simulink model "observador_mejorado"  (R2020a)
settings: Solver=ode45  StartTime=0.0  StopTime=25  MaxStep=1e-4  RelTol=1e-5
model workspace: external: MATLAB File D:\Ferran\Facultad\UNCuyo\Meca\Automática y Máquinas Eléctricas\Proyecto final\matlab2\parametros_y_especs\parametros_y_especif.m (data not in the file)
undefined symbols (not defined in the file): alpha_Cu, Ba, beq, Cts, Jeq, Ke_int, Ke_theta, Ke_theta_m, Ke_w, Ke_w_m, Ksa, Ksia, L_ls, lambda_m, Ld, Lq, Pp, r, R0, Rd, Rq, Rref, Rts_amb, sigbuilder_block, Tref
settings Model: Creator=Ferran  LastModifiedBy=Ferran

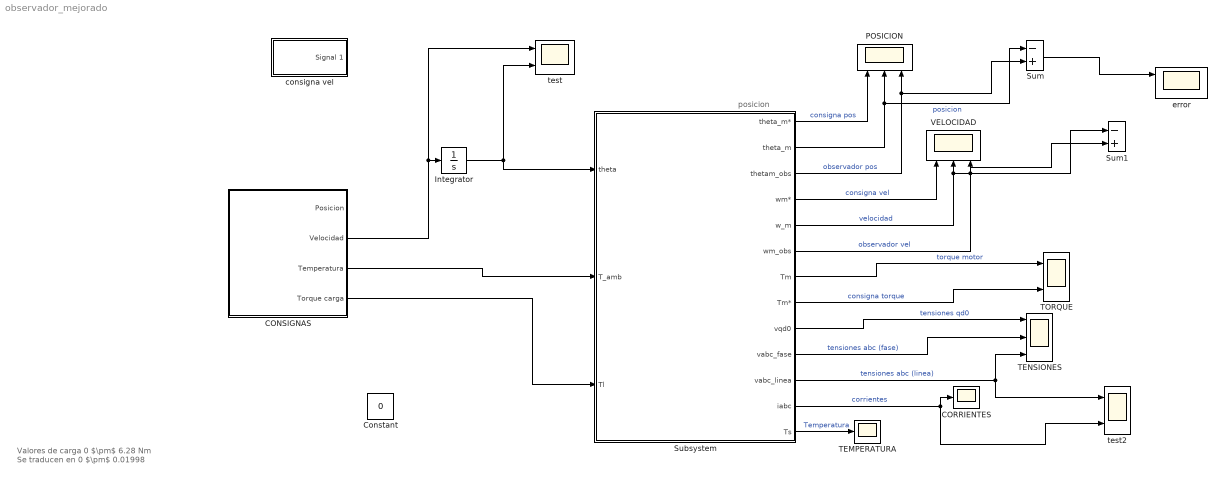
== system observador_mejorado ==
  note: posicion
  note: Valores de carga
      |
      | 0 $\pm$ 6.28 Nm
      | Se traducen en
      | 0 $\pm$ 0.01998
  CONSIGNAS : Subsystem  Tag=STV Subsys  LoadFcn=sigbuilder_block('load');  StartFcn=sigbuilder_block('start');  StopFcn=sigbuilder_block('stop');  ClipboardFcn=sigbuilder_block('clipboard');  mask(Sigbuilder block){tuvar=[0:10]}
      mask help: Simulink:masks:SigbuilderBlock_MD
      mask init:
      | if ~strcmp(get_param(bdroot(gcbh),'SimulationStatus'),'stopped') tuvar = sigbuilder_block('maskInit'); end
      settings: CopyFcn=sigbuilder_block('copy');  DeleteFcn=sigbuilder_block('delete');  ModelCloseFcn=sigbuilder_block('modelClose');  PreSaveFcn=sigbuilder_block('preSave');  PauseFcn=sigbuilder_block('pause');  ContinueFcn=sigbuilder_block('continue');  NameChangeFcn=sigbuilder_block('namechange');  OpenFcn=sigbuilder_block('open',[75 32.4 967.2 484.8 ]);  CloseFcn=sigbuilder_block('close');
      mask Display: plot(0, 0, 100, 100,[2, 2, 32, 32, 2], [68, 8, 8, 68, 68],[32, 2], [38, 38], [32, 19, 2],[53, 60, 44], [32, 17, 17, 2],[16, 16, 31, 31]);txt = getActiveGroup(gcbh);text(2, 100, txt,'verticalAlignment', 'top');
  CORRIENTES : Scope
  Constant : Constant  Value=0
  Integrator : Integrator
  POSICION : Scope  NumInputPorts=3
  Subsystem : Subsystem
  Sum : Sum  Inputs=-+
  Sum1 : Sum  Inputs=-+
  TEMPERATURA : Scope
  TENSIONES : Scope  NumInputPorts=3
  TORQUE : Scope  NumInputPorts=2
  VELOCIDAD : Scope  NumInputPorts=3
  consigna vel : Subsystem  Tag=STV Subsys  LoadFcn=sigbuilder_block('load');  StartFcn=sigbuilder_block('start');  StopFcn=sigbuilder_block('stop');  ClipboardFcn=sigbuilder_block('clipboard');  mask(Sigbuilder block){tuvar=[0:10]}
      mask help: Simulink:masks:SigbuilderBlock_MD
      mask init:
      | if ~strcmp(get_param(bdroot(gcbh),'SimulationStatus'),'stopped') tuvar = sigbuilder_block('maskInit'); end
      settings: CopyFcn=sigbuilder_block('copy');  DeleteFcn=sigbuilder_block('delete');  ModelCloseFcn=sigbuilder_block('modelClose');  PreSaveFcn=sigbuilder_block('preSave');  PauseFcn=sigbuilder_block('pause');  ContinueFcn=sigbuilder_block('continue');  NameChangeFcn=sigbuilder_block('namechange');  OpenFcn=sigbuilder_block('open',[5.4 0 1141.2 552.6 ]);  CloseFcn=sigbuilder_block('close');
      mask Display: plot(0, 0, 100, 100,[2, 2, 32, 32, 2], [68, 8, 8, 68, 68],[32, 2], [38, 38], [32, 19, 2],[53, 60, 44], [32, 17, 17, 2],[16, 16, 31, 31]);txt = getActiveGroup(gcbh);text(2, 100, txt,'verticalAlignment', 'top');
  error : Scope  NumInputPorts=2
  test : Scope  NumInputPorts=2
  test2 : Scope  NumInputPorts=2
  wires:
  CONSIGNAS/3(Temperatura) -> Subsystem/2(T_amb)
  Subsystem/2(theta_m) -> POSICION/2, Sum/1  "posicion"
  Subsystem/1(theta_m*) -> POSICION/1  "consigna pos"
  Subsystem/3(thetam_obs) -> POSICION/3, Sum/2  "observador pos"
  Subsystem/5(w_m) -> Sum1/1, VELOCIDAD/2  "velocidad"
  Subsystem/4(wm*) -> VELOCIDAD/1  "consigna vel"
  Subsystem/6(wm_obs) -> Sum1/2, VELOCIDAD/3  "observador vel"
  Subsystem/7(Tm) -> TORQUE/1  "torque motor"
  Subsystem/8(Tm*) -> TORQUE/2  "consigna torque"
  Subsystem/9(vqd0) -> TENSIONES/1  "tensiones qd0"
  Subsystem/10(vabc_fase) -> TENSIONES/2  "tensiones abc (fase)"
  Subsystem/12(iabc) -> CORRIENTES/1, test2/2  "corrientes"
  Subsystem/13(Ts) -> TEMPERATURA/1  "Temperatura"
  CONSIGNAS/2(Velocidad) -> test/1, Integrator/1
  Subsystem/11(vabc_linea) -> TENSIONES/3, test2/1  "tensiones abc (linea)"
  Integrator/1 -> test/2, Subsystem/1(theta)
  CONSIGNAS/4(Torque carga) -> Subsystem/3(Tl)
  Sum/1 -> error/1

== system observador_mejorado/CONSIGNAS ==
  Demux : Demux  Tag=STV Demux
      settings: DisplayOption=none
  FromWs : FromWorkspace  Tag=STV FromWs  VariableName=tuvar
      SigBuilderData=|
      | common.afterFinalStr = 'Extrapolate'
      | common.sampleTime = 0
      | dataSet.timeRange = [0 25]
      | dataSet.name = 'Group 1'
      | sbobj.Groups.Name = 'Group 1'
      | sbobj.Groups.Signals(1).Name = 'Posicion'
      | sbobj.Groups.Signals(1).XData = [0 5 10 15 20 25]
      | sbobj.Groups.Signals(1).YData = [0 0 6.28318530718 6.28318530718 0 0]
      | sbobj.Groups.Signals(2).Name = 'Velocidad'
      | sbobj.Groups.Signals(2).XData = [0 5 5.25 9.75 10 15 15.25 19.75 20 25]
      | sbobj.Groups.Signals(2).YData = [0 0 1.3228 1.3228 0 0 -1.3228 -1.3228 0 0]
      | sbobj.Groups.Signals(3).Name = 'Temperatura'
      | sbobj.Groups.Signals(3).XData = [0 25]
      | sbobj.Groups.Signals(3).YData = [40 40]
      | sbobj.Groups.Signals(4).Name = 'Torque carga'
      | sbobj.Groups.Signals(4).XData = [0 12.5 12.5 25]
      | sbobj.Groups.Signals(4).YData = [0 0 6.28 6.28]
      | sbobj.Groups.TimeRange = [0 25]
  Posicion : Outport  Tag=STV Outport
  Velocidad : Outport  Tag=STV Outport  Port=2
  Temperatura : Outport  Tag=STV Outport  Port=3
  Torque carga : Outport  Tag=STV Outport  Port=4
  wires:
  FromWs/1 -> Demux/1
  Demux/1 -> Posicion/1
  Demux/2 -> Velocidad/1
  Demux/3 -> Temperatura/1
  Demux/4 -> Torque carga/1

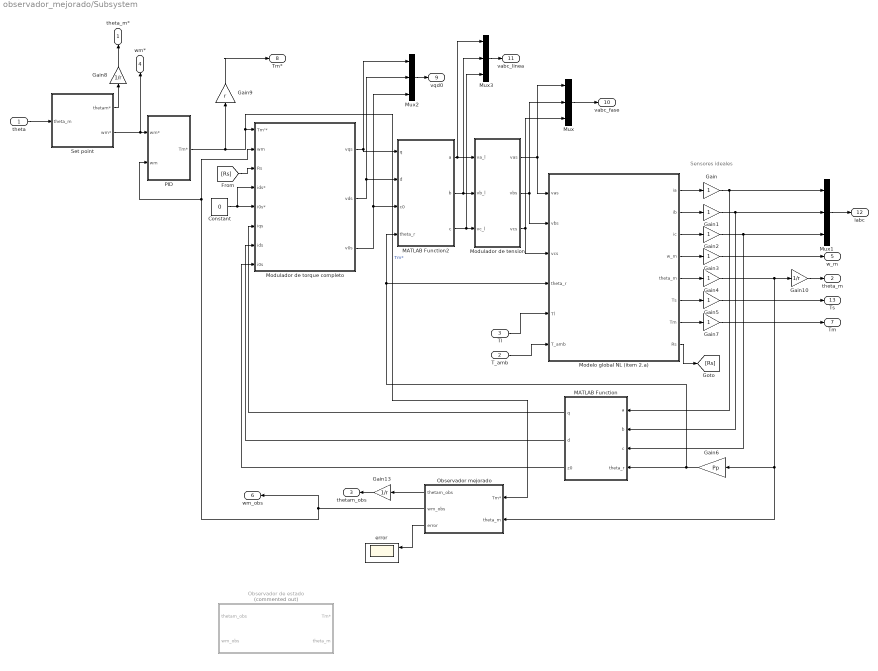
== system observador_mejorado/Subsystem ==
  note: Sensores ideales
  theta : Inport
  T_amb : Inport  Port=2
  Tl : Inport  Port=3
  Constant : Constant  Value=0
  Gain{,1..5,7} (7 alike) : Gain
  Gain10 : Gain  Gain=1/r
  Gain13 : Gain  Gain=1/r
  Gain6 : Gain  Gain=Pp
  Gain8 : Gain  Gain=1/r
  Gain9 : Gain  Gain=r
  MATLAB Function : MATLAB Function  TreatAsAtomicUnit=on
  MATLAB Function2 : MATLAB Function  TreatAsAtomicUnit=on
  Modelo global NL (item 2.a) : Subsystem
  Modulador de tension : Subsystem
  Modulador de torque completo : Subsystem
  Mux{,1..3} (4 alike) : Mux  Inputs=3
  Observador de estado : Subsystem  Commented=on
  Observador mejorado : Subsystem
  PID : Subsystem
  Set point : Subsystem
  error : Scope  NumInputPorts=2
  theta_m* : Outport
  theta_m : Outport  Port=2
  thetam_obs : Outport  Port=3
  wm* : Outport  Port=4
  w_m : Outport  Port=5
  wm_obs : Outport  Port=6
  Tm : Outport  Port=7
  Tm* : Outport  Port=8
  vqd0 : Outport  Port=9
  vabc_fase : Outport  Port=10
  vabc_linea : Outport  Port=11
  iabc : Outport  Port=12
  Ts : Outport  Port=13
  wires:
  Gain4/1 -> Gain10/1, Observador mejorado/2(theta_m), Gain6/1
  Gain1/1 -> Mux1/2, MATLAB Function/2(b)
  Gain/1 -> Mux1/1, MATLAB Function/1(a)
  Gain6/1 -> Modelo global NL (item 2.a)/4(theta_r), MATLAB Function2/4(theta_r), MATLAB Function/4(theta_r)
  MATLAB Function2/3(c) -> Modulador de tension/3(vc_l), Mux3/3
  Modelo global NL (item 2.a)/2(ib) -> Gain1/1
  Observador mejorado/1(thetam_obs) -> Gain13/1
  Modulador de torque completo/1(vqs) -> MATLAB Function2/1(q), Mux2/1
  Set point/1(thetam*) -> Gain8/1
  T_amb/1 -> Modelo global NL (item 2.a)/6(T_amb)
  MATLAB Function/3(z0) -> Modulador de torque completo/8(i0s)
  theta/1 -> Set point/1(theta_m)
  Modulador de tension/2(vbs) -> Modelo global NL (item 2.a)/2(vbs), Mux/2
  Modelo global NL (item 2.a)/5(theta_m) -> Gain4/1
  Modulador de tension/1(vas) -> Modelo global NL (item 2.a)/1(vas), Mux/1
  Tl/1 -> Modelo global NL (item 2.a)/5(Tl)
  Modelo global NL (item 2.a)/4(w_m) -> Gain3/1
  Modelo global NL (item 2.a)/1(ia) -> Gain/1
  Constant/1 -> Modulador de torque completo/4(ids*), Modulador de torque completo/5(i0s*)
  Gain2/1 -> Mux1/3, MATLAB Function/3(c)
  MATLAB Function/2(d) -> Modulador de torque completo/7(ids)
  Modulador de torque completo/2(vds) -> Mux2/2, MATLAB Function2/2(d)
  Gain7/1 -> Tm/1
  MATLAB Function/1(q) -> Modulador de torque completo/6(iqs)
  [Rs] -> Modulador de torque completo/3(Rs)
  Modulador de torque completo/3(v0s) -> Mux2/3, MATLAB Function2/3(c0)
  Gain5/1 -> Ts/1
  Modulador de tension/3(vcs) -> Modelo global NL (item 2.a)/3(vcs), Mux/3
  PID/1(Tm*) -> Gain9/1, Observador mejorado/1(Tm*), Modulador de torque completo/1(Tm'*)  "Tm*"
  Modelo global NL (item 2.a)/6(Ts) -> Gain5/1
  MATLAB Function2/2(b) -> Modulador de tension/2(vb_l), Mux3/2
  Modelo global NL (item 2.a)/3(ic) -> Gain2/1
  MATLAB Function2/1(a) -> Modulador de tension/1(va_l), Mux3/1
  Modelo global NL (item 2.a)/8(Rs) -> [Rs]
  Mux/1 -> vabc_fase/1
  Mux1/1 -> iabc/1
  Mux2/1 -> vqd0/1
  Modelo global NL (item 2.a)/7(Tm) -> Gain7/1
  Gain8/1 -> theta_m*/1
  Set point/2(wm*) -> wm*/1, PID/1(wm*)
  Gain3/1 -> w_m/1
  Gain10/1 -> theta_m/1
  Observador mejorado/2(wm_obs) -> Modulador de torque completo/2(wm), PID/2(wm), wm_obs/1
  Gain13/1 -> thetam_obs/1
  Gain9/1 -> Tm*/1
  Mux3/1 -> vabc_linea/1
  Observador mejorado/3(error) -> error/1

== system observador_mejorado/consigna vel ==
  Demux : Demux  Tag=STV Demux  Outputs=1
      settings: DisplayOption=none
  FromWs : FromWorkspace  Tag=STV FromWs  VariableName=tuvar
      SigBuilderData=|
      | common.afterFinalStr = 'Extrapolate'
      | common.sampleTime = 0
      | dataSet.timeRange = [0 25]
      | dataSet.name = 'Group 1'
      | sbobj.Groups.Name = 'Group 1'
      | sbobj.Groups.Signals.Name = 'Signal 1'
      | sbobj.Groups.Signals.XData = [0 5 7.5 10 15 16.25 18.75 20 25]
      | sbobj.Groups.Signals.YData = [0 0 1.68 0 0 -1.68 -1.68 0 0]
      | sbobj.Groups.TimeRange = [0 25]
  Signal 1 : Outport  Tag=STV Outport
  wires:
  Demux/1 -> Signal 1/1
  FromWs/1 -> Demux/1

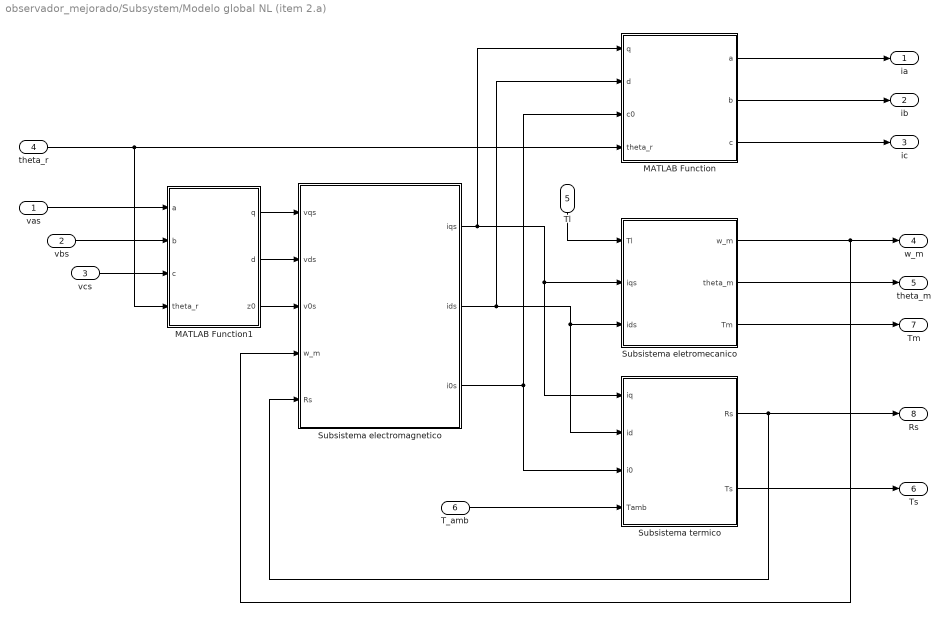
== system observador_mejorado/Subsystem/Modelo global NL (item 2.a) ==
  vas : Inport
  vbs : Inport  Port=2
  vcs : Inport  Port=3
  theta_r : Inport  Port=4
  Tl : Inport  Port=5
  T_amb : Inport  Port=6
  MATLAB Function : MATLAB Function  TreatAsAtomicUnit=on
  MATLAB Function1 : MATLAB Function  TreatAsAtomicUnit=on
  Subsistema electromagnetico : Subsystem
  Subsistema eletromecanico : Subsystem
  Subsistema termico : Subsystem
  ia : Outport
  ib : Outport  Port=2
  ic : Outport  Port=3
  w_m : Outport  Port=4
  theta_m : Outport  Port=5
  Ts : Outport  Port=6
  Tm : Outport  Port=7
  Rs : Outport  Port=8
  wires:
  Subsistema eletromecanico/1(w_m) -> Subsistema electromagnetico/4(w_m), w_m/1
  MATLAB Function1/1(q) -> Subsistema electromagnetico/1(vqs)
  Subsistema eletromecanico/2(theta_m) -> theta_m/1
  MATLAB Function/1(a) -> ia/1
  MATLAB Function/2(b) -> ib/1
  MATLAB Function1/2(d) -> Subsistema electromagnetico/2(vds)
  Subsistema electromagnetico/2(ids) -> Subsistema termico/2(id), Subsistema eletromecanico/3(ids), MATLAB Function/2(d)
  Tl/1 -> Subsistema eletromecanico/1(Tl)
  Subsistema termico/2(Ts) -> Ts/1
  Subsistema electromagnetico/3(i0s) -> Subsistema termico/3(i0), MATLAB Function/3(c0)
  Subsistema termico/1(Rs) -> Subsistema electromagnetico/5(Rs), Rs/1
  vbs/1 -> MATLAB Function1/2(b)
  vcs/1 -> MATLAB Function1/3(c)
  Subsistema electromagnetico/1(iqs) -> Subsistema termico/1(iq), Subsistema eletromecanico/2(iqs), MATLAB Function/1(q)
  vas/1 -> MATLAB Function1/1(a)
  MATLAB Function1/3(z0) -> Subsistema electromagnetico/3(v0s)
  MATLAB Function/3(c) -> ic/1
  Subsistema eletromecanico/3(Tm) -> Tm/1
  theta_r/1 -> MATLAB Function/4(theta_r), MATLAB Function1/4(theta_r)
  T_amb/1 -> Subsistema termico/4(Tamb)

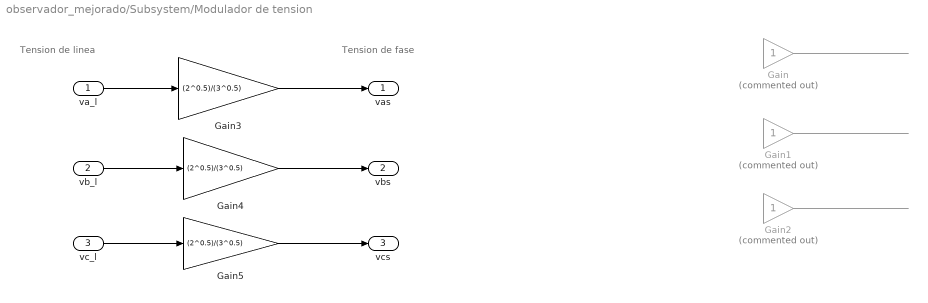
== system observador_mejorado/Subsystem/Modulador de tension ==
  note: Tension de fase
  note: Tension de linea
  va_l : Inport
  vb_l : Inport  Port=2
  vc_l : Inport  Port=3
  Gain : Gain  Commented=on
  Gain1 : Gain  Commented=on
  Gain2 : Gain  Commented=on
  Gain3 : Gain  Gain=(2^0.5)/(3^0.5)
  Gain4 : Gain  Gain=(2^0.5)/(3^0.5)
  Gain5 : Gain  Gain=(2^0.5)/(3^0.5)
  vas : Outport
  vbs : Outport  Port=2
  vcs : Outport  Port=3
  wires:
  Gain4/1 -> vbs/1
  Gain3/1 -> vas/1
  va_l/1 -> Gain3/1
  vb_l/1 -> Gain4/1
  vc_l/1 -> Gain5/1
  Gain5/1 -> vcs/1
  Gain1/1 -> ?
  ? -> Gain/1
  ? -> Gain2/1
  Gain2/1 -> ?
  ? -> Gain1/1
  Gain/1 -> ?

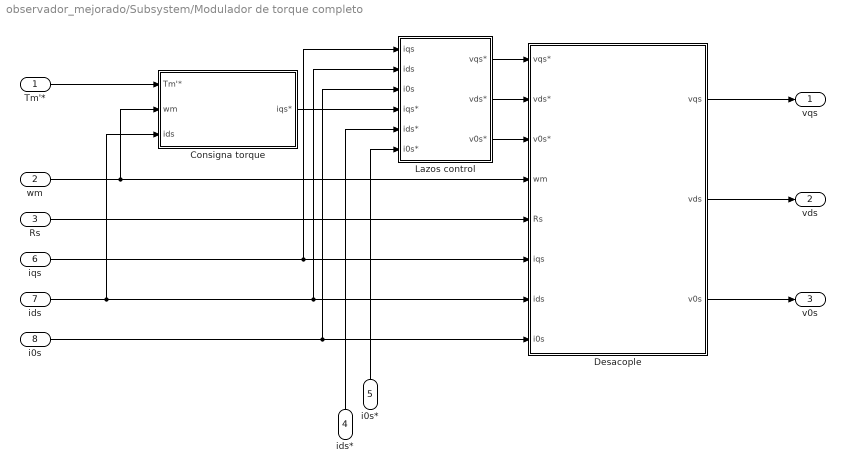
== system observador_mejorado/Subsystem/Modulador de torque completo ==
  Tm'* : Inport
  wm : Inport  Port=2
  Rs : Inport  Port=3
  ids* : Inport  Port=4
  i0s* : Inport  Port=5
  iqs : Inport  Port=6
  ids : Inport  Port=7
  i0s : Inport  Port=8
  Consigna torque : Subsystem
  Desacople : Subsystem
  Lazos control : Subsystem
  vqs : Outport
  vds : Outport  Port=2
  v0s : Outport  Port=3
  wires:
  ids/1 -> Consigna torque/3(ids), Desacople/7(ids), Lazos control/2(ids)
  Lazos control/3(v0s*) -> Desacople/3(v0s*)
  Rs/1 -> Desacople/5(Rs)
  Lazos control/1(vqs*) -> Desacople/1(vqs*)
  wm/1 -> Consigna torque/2(wm), Desacople/4(wm)
  i0s*/1 -> Lazos control/6(i0s*)
  Lazos control/2(vds*) -> Desacople/2(vds*)
  Consigna torque/1(iqs*) -> Lazos control/4(iqs*)
  i0s/1 -> Desacople/8(i0s), Lazos control/3(i0s)
  Desacople/2(vds) -> vds/1
  Tm'*/1 -> Consigna torque/1(Tm'*)
  iqs/1 -> Desacople/6(iqs), Lazos control/1(iqs)
  ids*/1 -> Lazos control/5(ids*)
  Desacople/3(v0s) -> v0s/1
  Desacople/1(vqs) -> vqs/1

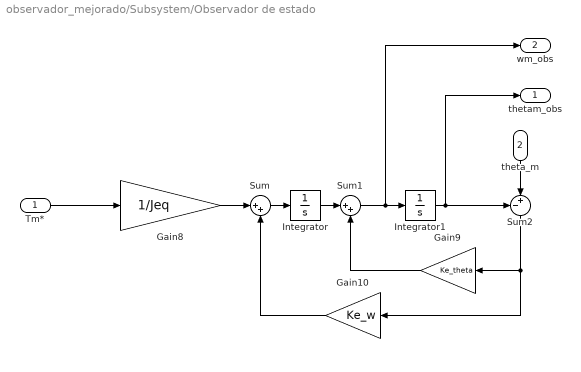
== system observador_mejorado/Subsystem/Observador de estado ==
  Tm* : Inport
  theta_m : Inport  Port=2
  Gain10 : Gain  Gain=Ke_w
  Gain8 : Gain  Gain=1/Jeq
  Gain9 : Gain  Gain=Ke_theta
  Integrator : Integrator
  Integrator1 : Integrator
  Sum : Sum  Inputs=|++
  Sum1 : Sum  Inputs=|++
  Sum2 : Sum  Inputs=-+|
  thetam_obs : Outport
  wm_obs : Outport  Port=2
  wires:
  Sum/1 -> Integrator/1
  Sum1/1 -> wm_obs/1, Integrator1/1
  Integrator1/1 -> thetam_obs/1, Sum2/1
  Gain9/1 -> Sum1/2
  Tm*/1 -> Gain8/1
  Gain8/1 -> Sum/1
  Integrator/1 -> Sum1/1
  Sum2/1 -> Gain10/1, Gain9/1
  Gain10/1 -> Sum/2
  theta_m/1 -> Sum2/2

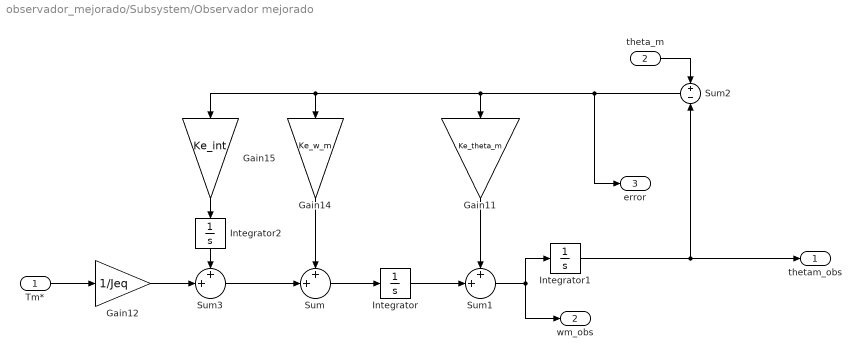
== system observador_mejorado/Subsystem/Observador mejorado ==
  Tm* : Inport
  theta_m : Inport  Port=2
  Gain11 : Gain  Gain=Ke_theta_m
  Gain12 : Gain  Gain=1/Jeq
  Gain14 : Gain  Gain=Ke_w_m
  Gain15 : Gain  Gain=Ke_int
  Integrator : Integrator
  Integrator1 : Integrator
  Integrator2 : Integrator
  Sum : Sum  Inputs=++|
  Sum1 : Sum  Inputs=++|
  Sum2 : Sum  Inputs=+-
  Sum3 : Sum  Inputs=++|
  thetam_obs : Outport
  wm_obs : Outport  Port=2
  error : Outport  Port=3
  wires:
  Sum/1 -> Integrator/1
  Sum1/1 -> wm_obs/1, Integrator1/1
  Integrator/1 -> Sum1/2
  Sum2/1 -> error/1, Gain11/1, Gain14/1, Gain15/1
  Gain12/1 -> Sum3/2
  theta_m/1 -> Sum2/1
  Gain15/1 -> Integrator2/1
  Sum3/1 -> Sum/2
  Gain14/1 -> Sum/1
  Tm*/1 -> Gain12/1
  Integrator1/1 -> thetam_obs/1, Sum2/2
  Gain11/1 -> Sum1/1
  Integrator2/1 -> Sum3/1

== system observador_mejorado/Subsystem/PID ==
  wm* : Inport
  wm : Inport  Port=2
  Gain10 : Gain  Gain=Ksia
  Gain8 : Gain  Gain=Ba
  Gain9 : Gain  Gain=Ksa
  Integrator : Integrator
  Integrator1 : Integrator
  Sum : Sum  Inputs=|+-
  Sum1 : Sum  Inputs=+++
  Tm* : Outport
  wires:
  Sum/1 -> Gain8/1, Integrator/1
  Gain9/1 -> Sum1/2
  wm*/1 -> Sum/1
  Integrator/1 -> Integrator1/1, Gain9/1
  Gain8/1 -> Sum1/3
  Gain10/1 -> Sum1/1
  wm/1 -> Sum/2
  Integrator1/1 -> Gain10/1
  Sum1/1 -> Tm*/1

== system observador_mejorado/Subsystem/Set point ==
  note: Referencia de posicion articular q
  theta_m : Inport
  Derivative : Derivative
  Gain8 : Gain  Gain=r
  thetam* : Outport
  wm* : Outport  Port=2
  wires:
  Derivative/1 -> wm*/1
  theta_m/1 -> Gain8/1
  Gain8/1 -> thetam*/1, Derivative/1

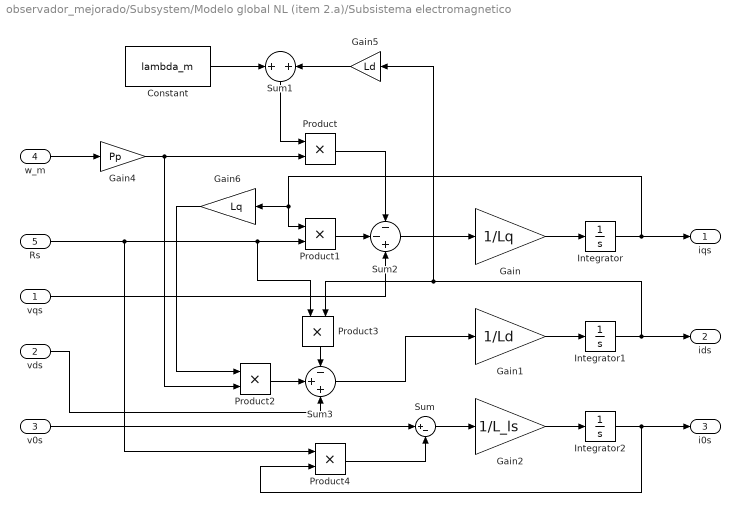
== system observador_mejorado/Subsystem/Modelo global NL (item 2.a)/Subsistema electromagnetico ==
  vqs : Inport
  vds : Inport  Port=2
  v0s : Inport  Port=3
  w_m : Inport  Port=4
  Rs : Inport  Port=5
  Constant : Constant  Value=lambda_m
  Gain : Gain  Gain=1/Lq
  Gain1 : Gain  Gain=1/Ld
  Gain2 : Gain  Gain=1/L_ls
  Gain4 : Gain  Gain=Pp
  Gain5 : Gain  Gain=Ld
  Gain6 : Gain  Gain=Lq
  Integrator : Integrator
  Integrator1 : Integrator
  Integrator2 : Integrator
  Product{,1..4} (5 alike) : Product
  Sum : Sum  Inputs=|+-
  Sum1 : Sum  Inputs=+|+
  Sum2 : Sum  Inputs=--+
  Sum3 : Sum  Inputs=-++
  iqs : Outport
  ids : Outport  Port=2
  i0s : Outport  Port=3
  wires:
  Sum2/1 -> Gain/1
  Integrator1/1 -> ids/1, Product3/2, Gain5/1
  Product1/1 -> Sum2/2
  Integrator/1 -> iqs/1, Gain6/1, Product1/1
  Sum3/1 -> Gain1/1
  Constant/1 -> Sum1/1
  Gain2/1 -> Integrator2/1
  Product3/1 -> Sum3/1
  Gain6/1 -> Product2/1
  Rs/1 -> Product1/2, Product3/1, Product4/1
  v0s/1 -> Sum/1
  w_m/1 -> Gain4/1
  Gain1/1 -> Integrator1/1
  Integrator2/1 -> i0s/1, Product4/2
  vqs/1 -> Sum2/3
  Product4/1 -> Sum/2
  Product2/1 -> Sum3/2
  Gain5/1 -> Sum1/2
  vds/1 -> Sum3/3
  Gain4/1 -> Product/2, Product2/2
  Sum1/1 -> Product/1
  Product/1 -> Sum2/1
  Gain/1 -> Integrator/1
  Sum/1 -> Gain2/1

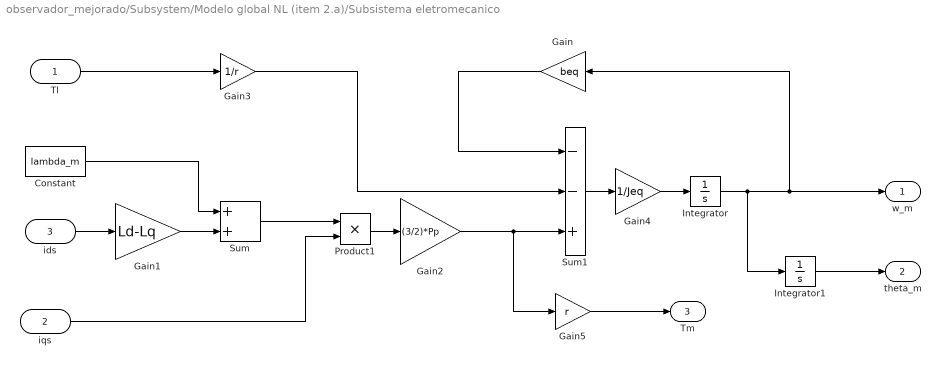
== system observador_mejorado/Subsystem/Modelo global NL (item 2.a)/Subsistema eletromecanico ==
  Tl : Inport
  iqs : Inport  Port=2
  ids : Inport  Port=3
  Constant : Constant  Value=lambda_m
  Gain : Gain  Gain=beq
  Gain1 : Gain  Gain=Ld-Lq
  Gain2 : Gain  Gain=(3/2)*Pp
  Gain3 : Gain  Gain=1/r
  Gain4 : Gain  Gain=1/Jeq
  Gain5 : Gain  Gain=r
  Integrator : Integrator
  Integrator1 : Integrator
  Product1 : Product
  Sum : Sum
  Sum1 : Sum  Inputs=--+
  w_m : Outport
  theta_m : Outport  Port=2
  Tm : Outport  Port=3
  wires:
  Gain1/1 -> Sum/2
  Constant/1 -> Sum/1
  Gain/1 -> Sum1/1
  Product1/1 -> Gain2/1
  Tl/1 -> Gain3/1
  ids/1 -> Gain1/1
  Sum1/1 -> Gain4/1
  Gain4/1 -> Integrator/1
  Integrator/1 -> w_m/1, Gain/1, Integrator1/1
  Gain3/1 -> Sum1/2
  iqs/1 -> Product1/2
  Integrator1/1 -> theta_m/1
  Sum/1 -> Product1/1
  Gain2/1 -> Gain5/1, Sum1/3
  Gain5/1 -> Tm/1

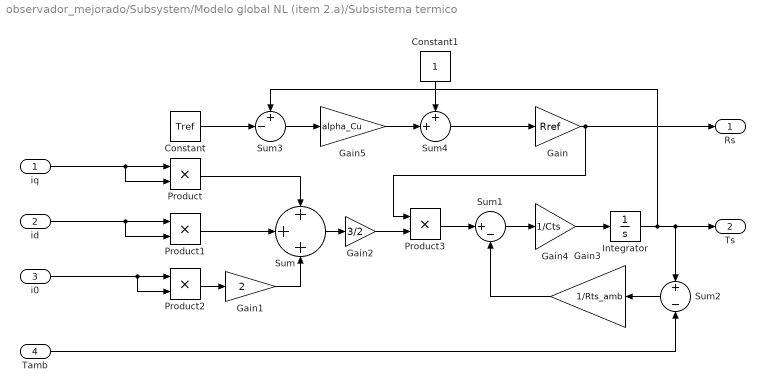
== system observador_mejorado/Subsystem/Modelo global NL (item 2.a)/Subsistema termico ==
  iq : Inport
  id : Inport  Port=2
  i0 : Inport  Port=3
  Tamb : Inport  Port=4
  Constant : Constant  Value=Tref
  Constant1 : Constant
  Gain : Gain  Gain=Rref
  Gain1 : Gain  Gain=2
  Gain2 : Gain  Gain=3/2
  Gain3 : Gain  Gain=1/Rts_amb
  Gain4 : Gain  Gain=1/Cts
  Gain5 : Gain  Gain=alpha_Cu
  Integrator : Integrator  InitialCondition=40
  Product{,1..3} (4 alike) : Product
  Sum : Sum  Inputs=+++
  Sum1 : Sum  Inputs=|+-
  Sum2 : Sum  Inputs=+-
  Sum3 : Sum  Inputs=+-|
  Sum4 : Sum  Inputs=++|
  Rs : Outport
  Ts : Outport  Port=2
  wires:
  Product2/1 -> Gain1/1
  Product/1 -> Sum/1
  id/1 -> Product1/1, Product1/2
  iq/1 -> Product/1, Product/2
  Sum4/1 -> Gain/1
  Sum3/1 -> Gain5/1
  Gain/1 -> Product3/1, Rs/1
  Constant1/1 -> Sum4/1
  Sum1/1 -> Gain4/1
  Gain3/1 -> Sum1/2
  Gain4/1 -> Integrator/1
  Product3/1 -> Sum1/1
  Sum2/1 -> Gain3/1
  i0/1 -> Product2/1, Product2/2
  Sum/1 -> Gain2/1
  Product1/1 -> Sum/2
  Tamb/1 -> Sum2/2
  Constant/1 -> Sum3/2
  Gain5/1 -> Sum4/2
  Integrator/1 -> Sum3/1, Sum2/1, Ts/1
  Gain1/1 -> Sum/3
  Gain2/1 -> Product3/2

== system observador_mejorado/Subsystem/Modulador de torque completo/Consigna torque ==
  note: Consigna de torque
  Tm'* : Inport
  wm : Inport  Port=2
  ids : Inport  Port=3
  Constant : Constant  Value=lambda_m
  Divide : Product  Inputs=*/
  Gain1 : Gain  Gain=beq
  Gain2 : Gain  Gain=(Ld-Lq)
  Gain3 : Gain  Gain=(3/2)*Pp
  Sum : Sum
  Sum1 : Sum
  iqs* : Outport
  wires:
  Constant/1 -> Sum1/2
  Gain2/1 -> Sum1/1
  Tm'*/1 -> Sum/1
  Divide/1 -> iqs*/1
  Sum1/1 -> Gain3/1
  Gain3/1 -> Divide/2
  Gain1/1 -> Sum/2
  Sum/1 -> Divide/1
  wm/1 -> Gain1/1
  ids/1 -> Gain2/1

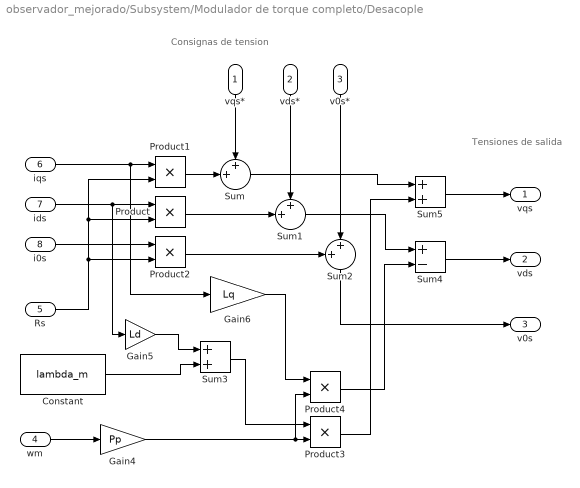
== system observador_mejorado/Subsystem/Modulador de torque completo/Desacople ==
  note: Tensiones
      | de salida
  note: Consignas de tension
  vqs* : Inport
  vds* : Inport  Port=2
  v0s* : Inport  Port=3
  wm : Inport  Port=4
  Rs : Inport  Port=5
  iqs : Inport  Port=6
  ids : Inport  Port=7
  i0s : Inport  Port=8
  Constant : Constant  Value=lambda_m
  Gain4 : Gain  Gain=Pp
  Gain5 : Gain  Gain=Ld
  Gain6 : Gain  Gain=Lq
  Product{,1..4} (5 alike) : Product
  Sum : Sum  Inputs=++|
  Sum1 : Sum  Inputs=++|
  Sum2 : Sum  Inputs=++|
  Sum3 : Sum
  Sum4 : Sum  Inputs=+-
  Sum5 : Sum
  vqs : Outport
  vds : Outport  Port=2
  v0s : Outport  Port=3
  wires:
  Sum/1 -> Sum5/1
  Sum5/1 -> vqs/1
  iqs/1 -> Product1/1, Gain6/1
  Product2/1 -> Sum2/1
  ids/1 -> Product/1, Gain5/1
  Gain4/1 -> Product4/2, Product3/2
  Product3/1 -> Sum5/2
  Rs/1 -> Product2/2, Product/2, Product1/2
  Product1/1 -> Sum/2
  Sum2/1 -> v0s/1
  Sum4/1 -> vds/1
  Constant/1 -> Sum3/2
  Gain5/1 -> Sum3/1
  Sum1/1 -> Sum4/1
  i0s/1 -> Product2/1
  Product4/1 -> Sum4/2
  Sum3/1 -> Product3/1
  wm/1 -> Gain4/1
  Product/1 -> Sum1/2
  Gain6/1 -> Product4/1
  v0s*/1 -> Sum2/2
  vds*/1 -> Sum1/1
  vqs*/1 -> Sum/1

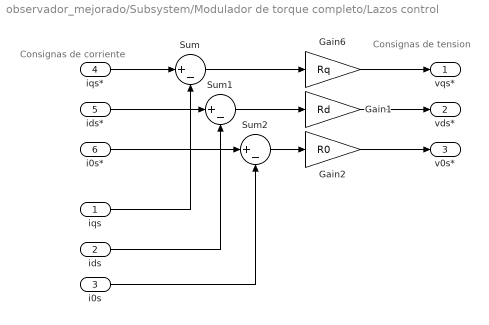
== system observador_mejorado/Subsystem/Modulador de torque completo/Lazos control ==
  note: Consignas de tension
  note: Consignas
      | de
      | corriente
  iqs : Inport
  ids : Inport  Port=2
  i0s : Inport  Port=3
  iqs* : Inport  Port=4
  ids* : Inport  Port=5
  i0s* : Inport  Port=6
  Gain1 : Gain  Gain=Rd
  Gain2 : Gain  Gain=R0
  Gain6 : Gain  Gain=Rq
  Sum : Sum  Inputs=|+-
  Sum1 : Sum  Inputs=|+-
  Sum2 : Sum  Inputs=|+-
  vqs* : Outport
  vds* : Outport  Port=2
  v0s* : Outport  Port=3
  wires:
  i0s*/1 -> Sum2/1
  i0s/1 -> Sum2/2
  Sum1/1 -> Gain1/1
  Gain6/1 -> vqs*/1
  Sum/1 -> Gain6/1
  Sum2/1 -> Gain2/1
  Gain1/1 -> vds*/1
  iqs*/1 -> Sum/1
  ids/1 -> Sum1/2
  iqs/1 -> Sum/2
  Gain2/1 -> v0s*/1
  ids*/1 -> Sum1/1

== matlab function observador_mejorado/Subsystem/Modelo global NL (item 2.a)/MATLAB Function1 ==
  data: a input; q output; b input; c input; theta_r input; d output; z0 output
function [q,d,z0] = TPark_directa(a,b,c,theta_r)
    fabc = [a;b;c];
    T = (2/3) * ...
        [ cos(theta_r) cos(theta_r - (2*pi)/3) cos(theta_r + (2*pi)/3);
        sin(theta_r) sin(theta_r - (2*pi)/3) sin(theta_r + (2*pi)/3);
        1/2                   1/2                  1/2];
  
  fqd0 = T*fabc;
  q = fqd0(1);
  d = fqd0(2);
  z0 = fqd0(3);
end

== matlab function observador_mejorado/Subsystem/Modelo global NL (item 2.a)/MATLAB Function ==
  data: q input; a output; d input; c0 input; theta_r input; b output; c output
function [a,b,c] = TPark_inversa(q,d,c0,theta_r)
    fqd0 = [q;d;c0];
    T = [cos(theta_r)               sin(theta_r)            1;
        cos(theta_r - (2*pi)/3)    sin(theta_r - (2*pi)/3) 1;
        cos(theta_r + (2*pi)/3)    sin(theta_r + (2*pi)/3) 1];
    
    fabc = T*fqd0;
    
    a = fabc(1);
    b = fabc(2);
    c = fabc(3);
end

== matlab function observador_mejorado/Subsystem/MATLAB Function ==
  data: a input; q output; b input; c input; theta_r input; d output; z0 output
function [q,d,z0] = TPark_directa(a,b,c,theta_r)
    fabc = [a;b;c];
    T = (2/3) * ...
        [ cos(theta_r) cos(theta_r - (2*pi)/3) cos(theta_r + (2*pi)/3);
        sin(theta_r) sin(theta_r - (2*pi)/3) sin(theta_r + (2*pi)/3);
        1/2                   1/2                  1/2];
  
  fqd0 = T*fabc;
  q = fqd0(1);
  d = fqd0(2);
  z0 = fqd0(3);
end

== matlab function observador_mejorado/Subsystem/MATLAB Function2 ==
  data: q input; a output; d input; c0 input; theta_r input; b output; c output
function [a,b,c] = TPark_inversa(q,d,c0,theta_r)
    fqd0 = [q;d;c0];
    T = [cos(theta_r)               sin(theta_r)            1;
        cos(theta_r - (2*pi)/3)    sin(theta_r - (2*pi)/3) 1;
        cos(theta_r + (2*pi)/3)    sin(theta_r + (2*pi)/3) 1];
    
    fabc = T*fqd0;
    
    a = fabc(1);
    b = fabc(2);
    c = fabc(3);
end
